simulink model "kalmanovFilter"  (R2013b)
settings: Solver=ode45  StartTime=0.0  StopTime=100.0  RelTol=1e-3
values from neighbouring files (symbols this model uses):
  A = [-1/8 1/8 0 0; 0 -1/10 1/10 0;0 0 -1/1.2 1/1.2; 0 0 0 -1/0.8]    [Parametri.m]
  B = [0; 0; 0; 1/0.8]    [Parametri.m]
  C = [1 0 0 0]    [Parametri.m]
  D = 0    [Parametri.m]
libraries: commnoisgen2 x2
settings Model: Creator=sadzi  LastModifiedBy=sadzi

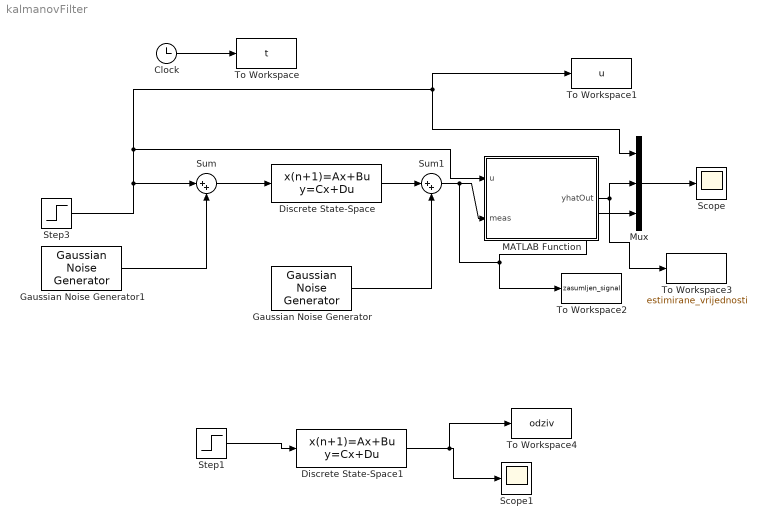
== system kalmanovFilter ==
  Clock : Clock
  Discrete State-Space : DiscreteStateSpace  A=A  B=B  C=C  D=D
  Discrete State-Space1 : DiscreteStateSpace  A=A  B=B  C=C  D=D
  Gaussian Noise Generator : commnoisgen2/Gaussian Noise Generator  m=0  d=R  s=1  Ts=0.1  frameBased=off  sampPerFrame=1  orient=off  outDataType=double
  Gaussian Noise Generator1 : commnoisgen2/Gaussian Noise Generator  m=0  d=0.01^2  s=1  Ts=1  frameBased=off  sampPerFrame=1  orient=off  outDataType=double
  MATLAB Function : MATLAB Function  TreatAsAtomicUnit=on
  Mux : Mux  Inputs=3
  Scope : Scope
  Scope1 : Scope
  Step1 : Step  Time=0.5  SampleTime=0
  Step3 : Step  Time=0.5  SampleTime=0
  Sum : Sum  Inputs=|++
  Sum1 : Sum  Inputs=|++
  To Workspace : ToWorkspace  VariableName=t  SampleTime=-1
  To Workspace1 : ToWorkspace  VariableName=u  SampleTime=-1
  To Workspace2 : ToWorkspace  VariableName=zasumljen_signal  SampleTime=-1
  To Workspace3 : ToWorkspace  VariableName=estimirane_vrijednosti  SampleTime=-1
  To Workspace4 : ToWorkspace  VariableName=odziv  SampleTime=-1
  wires:
  Step3/1 -> Sum/1, MATLAB Function/1(u), Mux/1, To Workspace1/1
  Discrete State-Space/1 -> Sum1/1
  Sum/1 -> Discrete State-Space/1
  Sum1/1 -> Mux/3, To Workspace2/1, MATLAB Function/2(meas)
  MATLAB Function/1(yhatOut) -> Mux/2, To Workspace3/1
  Mux/1 -> Scope/1
  Gaussian Noise Generator1/1 -> Sum/2
  Gaussian Noise Generator/1 -> Sum1/2
  Clock/1 -> To Workspace/1
  Step1/1 -> Discrete State-Space1/1
  Discrete State-Space1/1 -> To Workspace4/1, Scope1/1

== matlab function kalmanovFilter/MATLAB Function ==
  data: u input; meas input; yhatOut output
function yhatOut  = KALMAN(u,meas)

persistent P xhat A B C Q R
if isempty(P)
% Inicijalizacija prvi put
   xhat = [0;0];
   P = [1 0; 0 1];
   A=[-0.5 -0.7; 0.7 0];    
   B=[1;0];
   C=[2 6.5];
   Q = [0.01^2 0;0 0.01^2];
   R = 0.1^2;
end
% Racunanje estimiranog stanja i kovarijanse:
xhat = A*xhat + B*u;
P = A*P*A' + Q;
% Racunanje K
K = (P*C')/(C*P*C' + R);
% racunanje residuala
resid = meas - C*xhat;
% ažuraranje stanja
xhat = xhat + K*resid;
P = (eye(size(K,1))-K*C)*P;
% novi rezultati
xhatOut = xhat;
yhatOut = C*xhatOut;
